simulink model "MicrogridControl"  (R2025b)
settings: Solver=VariableStepAuto  StartTime=0.0  StopTime=8  FixedStep=Ts  RelTol=1e-3
PreLoadFcn:
  | NormalOperation;
  | MicrogridControlParam;
undefined symbols (not defined in the file): base, bessModeInitial, bessSystem, bessVoltage, breakerStatus, DiscIntNeverNeededParam, ee_sli_rtmsupport, event, gcbh, generator, gflInverter, gfmInverter, Inertia, lineInductance, lineResistance, machine, plannedIsland, pmsm, powerLimit, powerQuality, PV, PVInverter, ref, resync, solar, solarInsolationChange, systemFrequency, Ts, windController, windSystem, windTurbine
libraries: nesl_utility x234, ee_lib x174, fl_lib x143, eeGeneralControl x137, simulink x78, eeTransforms x47, slpidlib x23, nesl_utility_internal x12, eePwmGenerator x9, eeSinusoidalMeasurementV2 x9, custom_lib x7, batteryecm_lib x6
(part 23 of 25)

== system MicrogridControl/BESS/BESS Integrated3/Detailed/BESS Controller/Grid Forming/Measurement/Frequency Measurement/Frequency Measurement/Postive Sequence ==
  abc : Inport
  Complex to Real-Imag : ComplexToRealImag
  Demux : Demux  Outputs=3
  Symmetrical-Components Transform : eeTransforms/Symmetrical-Components Transform  PowerInvariant=off
  Terminator : Terminator
  Terminator1 : Terminator
  Terminator2 : Terminator
  Transpose : Math  Operator=transpose
  posSeq : Outport
  wires:
  Demux/3 -> Terminator2/1
  Demux/2 -> Terminator1/1
  Complex to Real-Imag/2 -> Terminator/1
  abc/1 -> Transpose/1
  Demux/1 -> Complex to Real-Imag/1
  Complex to Real-Imag/1 -> posSeq/1
  Symmetrical-Components Transform/1 -> Demux/1
  Transpose/1 -> Symmetrical-Components Transform/1

== system MicrogridControl/BESS/BESS Integrated3/Detailed/BESS Controller/Grid Forming/Power Control/ActivePowerControl/vsmControl/Damping Frequency ==
  fref : Inport
  ConstantFreqReference : Subsystem  VariantControl=constFreq
  WithFrequencyMeasurement : Subsystem  VariantControl=freqMeas
  fmeas : Outport

== system MicrogridControl/BESS/BESS Integrated3/Detailed/BESS Controller/Grid Forming/Power Control/ActivePowerControl/vsmControl/Power Reference Selection ==
  cntrlflag : Inport
  Pref : Inport  Port=2
  fref : Inport  Port=3
  Wsm : Inport  Port=4
  If : If
  If Action Subsystem : Subsystem  TreatAsAtomicUnit=on
  If Action Subsystem1 : Subsystem  TreatAsAtomicUnit=on
  Merge : Merge
  Scope : Scope
      settings: ActiveDisplayYMinimum=-0.024489680768438882  ActiveDisplayYMaximum=0.022000264002839637
  power : Outport
  wires:
  Wsm/1 -> [Wsm]
  Merge/1 -> power/1, Scope/1
  cntrlflag/1 -> If/1
  If/2 -> If Action Subsystem1/Action
  If Action Subsystem/1(Power) -> Merge/1
  [Wsm] -> If Action Subsystem/2(Wsm)
  fref/1 -> If Action Subsystem1/1(fref)
  [Wsm] -> If Action Subsystem1/2(Wsm)
  Pref/1 -> If Action Subsystem/1(Pref)
  If/1 -> If Action Subsystem/Action
  If Action Subsystem1/1(Power) -> Merge/2

== system MicrogridControl/BESS/BESS Integrated3/Detailed/BESS Controller/Grid Forming/Power Control/ReactiveControl/Voltage  Reference Selection/If Action Subsystem ==
  note: Vs-delV
  Qref : Inport
  Qmeas : Inport  Port=2
  Action Port : ActionPort  ActionPortLabel=if(u1 > 0)
  Constant : Constant  Value=voltreference
  Gain : Gain  Gain=1%QVoltDroop
  Low-Pass Filter (Discrete or Continuous) : eeGeneralControl/Low-Pass Filter (Discrete or Continuous)  K=1  T=QVoltFilterTC  B=inf  A=-inf  init_option=Specify as parameter  x0=0  Ts=activePowerSampleTime
  Product1 : Product
  Scope : Scope
      settings: ActiveDisplayYMinimum=-0.48916032129163395  ActiveDisplayYMaximum=3.1082432095983168
  Scope1 : Scope  NumInputPorts=2
      settings: ActiveDisplayYMinimum=-1.3317089011874013  ActiveDisplayYMaximum=1.2590787667985386  DataLoggingVariableName=ScopeData5
  Sum : Sum  Inputs=|+-
  Sum1 : Sum  Inputs=|++
  Vd : Outport
  wires:
  Product1/1 -> Vd/1  "V"
  Sum1/1 -> Product1/1
  Sum/1 -> Gain/1
  Low-Pass Filter (Discrete or Continuous)/1 -> Sum/2
  Qref/1 -> Scope1/1, Sum/1
  Gain/1 -> Sum1/1, Scope/1
  Qmeas/1 -> Scope1/2, Low-Pass Filter (Discrete or Continuous)/1
  Constant/1 -> Sum1/2, Product1/2

== system MicrogridControl/BESS/BESS Integrated3/Detailed/BESS Controller/Grid Forming/Power Control/ReactiveControl/Voltage  Reference Selection/If Action Subsystem1 ==
  note: Vs-delV
  Vref : Inport
  Vmeas : Inport  Port=2
  Action Port : ActionPort  ActionPortLabel=else
  Constant : Constant  Value=voltreference+0.05
  Gain : Gain  Gain=2%2/QVoltDroop
  Low-Pass Filter (Discrete or Continuous) : eeGeneralControl/Low-Pass Filter (Discrete or Continuous)  K=1  T=QVoltFilterTC  B=inf  A=-inf  init_option=Specify as parameter  x0=0  Ts=activePowerSampleTime
  Product1 : Product
  Scope : Scope
      settings: ActiveDisplayYMinimum=0.18931616111927707  ActiveDisplayYMaximum=6.6456315376534141  DataLoggingVariableName=ScopeData11  DataLoggingSaveFormat=Array
  Scope1 : Scope
      settings: ActiveDisplayYMinimum=-0.70570607622731063  ActiveDisplayYMaximum=1.2282506152075161  DataLoggingVariableName=ScopeData12  DataLoggingSaveFormat=Array
  Scope2 : Scope  NumInputPorts=2
      settings: ActiveDisplayYMinimum=-1  ActiveDisplayYMaximum=1  DataLoggingVariableName=ScopeData13  DataLoggingSaveFormat=Array
  Sum : Sum  Inputs=|+-
  Sum1 : Sum  Inputs=|++
  Voltage : Outport
  wires:
  Sum1/1 -> Product1/2
  Product1/1 -> Scope/1, Voltage/1  "V"
  Sum/1 -> Gain/1
  Low-Pass Filter (Discrete or Continuous)/1 -> Scope1/1, Sum/2
  Constant/1 -> Sum1/2
  Vmeas/1 -> Low-Pass Filter (Discrete or Continuous)/1, Scope2/2
  Gain/1 -> Sum1/1
  Vref/1 -> Sum/1, Product1/1, Scope2/1

== system MicrogridControl/Solar/Solar Plant Integrated/Detailed/PV Plant & Controller/Controller/MPPT/Solar PV Controller/DC voltage controller & current reference/Current limits ==
  Imax : Inport
  idref : Inport  Port=2
  Sqrt1 : Sqrt
  Square3 : Math  Operator=square
  Square4 : Math  Operator=square
  Sum9 : Sum  Inputs=|+-
  iubd : Outport
  iubq : Outport  Port=2
  wires:
  idref/1 -> Square4/1
  Sqrt1/1 -> iubq/1
  Imax/1 -> Square3/1, iubd/1
  Square4/1 -> Sum9/2
  Square3/1 -> Sum9/1
  Sum9/1 -> Sqrt1/1

== system MicrogridControl/Solar/Solar Plant Integrated/Detailed/PV Plant & Controller/Controller/MPPT/Solar PV Controller/DC voltage controller & current reference/If Action Subsystem ==
  note: id_ref_generator
  note: iq_ref_generator
  Q ref : Inport
  Vmag : Inport  Port=2
  P pv : Inport  Port=3
  vdc : Inport  Port=4
  vdc ref : Inport  Port=5
  Action Port : ActionPort
  Subsystem : Subsystem
  Subsystem1 : Subsystem
  iq ref : Outport
  id ref : Outport  Port=2
  wires:
  Subsystem/1(iqref) -> iq ref/1
  Subsystem1/1(idref) -> id ref/1
  vdc ref/1 -> Subsystem1/4(vdc ref)
  Vmag/1 -> Subsystem/1(V mag), Subsystem1/1(Vmag)
  vdc/1 -> Subsystem1/3(vdc)
  Q ref/1 -> Subsystem/3(Q ref)
  P pv/1 -> Subsystem1/2(P pv)
  [ubiq] -> Subsystem/2(iq ub)
  [ubid] -> Subsystem1/5(id ub)

== system MicrogridControl/Solar/Solar Plant Integrated/Detailed/PV Plant & Controller/Controller/MPPT/Solar PV Controller/DC voltage controller & current reference/Subsystem ==
  V mag : Inport
  iq ub : Inport  Port=2
  Q ref : Inport  Port=3
  Constant : Constant  Value=1e-3
  Data Type Conversion Inherited : simulink/Signal Attributes/Data Type Conversion Inherited  ConvertRealWorld=Real World Value  DoSatur=off
  Divide2 : Product  Inputs=*/
  Gain1 : Gain  Gain=-1
  Gain3 : Gain  Gain=-1
  Saturation Dynamic2 : simulink/Discontinuities/Saturation Dynamic  OutMin=[]  OutMax=[]  OutDataTypeStr=Inherit: Same as second input  OutDataType=fixdt(1, 16)  OutScaling=2^-10  DoSatur=off
  Scope : Scope  NumInputPorts=3
      settings: ActiveDisplayYMinimum=-1  ActiveDisplayYMaximum=1  DataLoggingVariableName=ScopeData8
  Switch : Switch  Criteria=u2 ~= 0  SaturateOnIntegerOverflow=off  InputSameDT=off
  iq ub1 : InportShadow  Port=2
  iqref : Outport
  wires:
  Gain1/1 -> iqref/1
  Data Type Conversion Inherited/1 -> Switch/3
  Constant/1 -> Data Type Conversion Inherited/2
  Switch/1 -> Divide2/2
  V mag/1 -> Switch/1, Switch/2, Data Type Conversion Inherited/1
  Saturation Dynamic2/1 -> Gain1/1
  iq ub/1 -> Scope/1, Saturation Dynamic2/1
  Gain3/1 -> Scope/3, Saturation Dynamic2/3
  Q ref/1 -> Divide2/1
  Divide2/1 -> Scope/2, Saturation Dynamic2/2
  iq ub1/1 -> Gain3/1

== system MicrogridControl/Solar/Solar Plant Integrated/Detailed/PV Plant & Controller/Controller/MPPT/Solar PV Controller/DC voltage controller & current reference/Subsystem1 ==
  Vmag : Inport
  P pv : Inport  Port=2
  vdc : Inport  Port=3
  vdc ref : Inport  Port=4
  id ub : Inport  Port=5
  Constant : Constant  Value=1e-3
  Constant4 : Constant  Value=0
  Data Type Conversion Inherited : simulink/Signal Attributes/Data Type Conversion Inherited  ConvertRealWorld=Real World Value  DoSatur=off
  Divide : Product  Inputs=/*
  Gain4 : Gain  Gain=1/(mVAbase)
  Saturation Dynamic1 : simulink/Discontinuities/Saturation Dynamic  OutMin=[]  OutMax=[]  OutDataTypeStr=Inherit: Same as second input  OutDataType=fixdt(1, 16)  OutScaling=2^-10  DoSatur=off
  Scope : Scope  NumInputPorts=2
      settings: ActiveDisplayYMinimum=961.255553355759  ActiveDisplayYMaximum=1181.2786383151777
  Scope1 : Scope  NumInputPorts=3
      settings: ActiveDisplayYMinimum=-1  ActiveDisplayYMaximum=1  DataLoggingVariableName=ScopeData7
  Sum : Sum  Inputs=|++
  Switch : Switch  Criteria=u2 ~= 0  SaturateOnIntegerOverflow=off  InputSameDT=off
  V_dc_Controller1 : Subsystem
  idref : Outport
  wires:
  Data Type Conversion Inherited/1 -> Switch/3
  Constant/1 -> Data Type Conversion Inherited/2
  Switch/1 -> Divide/1
  Vmag/1 -> Switch/1, Switch/2, Data Type Conversion Inherited/1
  vdc/1 -> Scope/1, V_dc_Controller1/1(vdc)
  Saturation Dynamic1/1 -> Scope1/3, idref/1
  Divide/1 -> Sum/1
  Gain4/1 -> Divide/2
  id ub/1 -> Saturation Dynamic1/1, Scope1/1
  vdc ref/1 -> Scope/2, V_dc_Controller1/2(vdc ref)
  Sum/1 -> Scope1/2, Saturation Dynamic1/2
  V_dc_Controller1/1(Out1) -> Sum/2
  P pv/1 -> Gain4/1
  Constant4/1 -> Saturation Dynamic1/3

== system MicrogridControl/Solar/Solar Plant Integrated/Detailed/PV Plant & Controller/Controller/MPPT/Solar PV Controller/PLL & Measurements/Subsystem ==
  abc : Inport
  Demux : Demux  Outputs=3
  Park Transform : eeTransforms/Park Transform  AxisAlignment=Q-axis  PowerInvariant=off
  "Sinusoidal Measurement (PLL, Three-Phase)" : eeSinusoidalMeasurementV2/Sinusoidal Measurement (PLL, Three-Phase)  InputFilter=on  InputNormalization=off  Kp_LF=Kppll  Ki_LF=Kipll  F0=frequency  Theta0=initialPhase  Ts=sampleTime
  Terminator : Terminator
  mag : Outport
  freq : Outport  Port=2
  angle : Outport  Port=3
  Vd : Outport  Port=4
  Vq : Outport  Port=5
  wires:
  "Sinusoidal Measurement (PLL, Three-Phase)"/3 -> mag/1
  "Sinusoidal Measurement (PLL, Three-Phase)"/1 -> freq/1
  Demux/2 -> Vq/1
  Demux/1 -> Vd/1
  Park Transform/1 -> Demux/1
  abc/1 -> "Sinusoidal Measurement (PLL, Three-Phase)"/1, Park Transform/1
  Demux/3 -> Terminator/1
  "Sinusoidal Measurement (PLL, Three-Phase)"/2 -> Park Transform/2, angle/1

== system MicrogridControl/Solar/Solar Plant Integrated/Detailed/PV Plant & Controller/Controller/MPPT/Solar PV Controller/Variant Subsystem/INC MPP ==
  Ipv : Inport
  Vpv : Inport  Port=2
  Abs : Abs  SaturateOnIntegerOverflow=off
  Add : Sum
  Constant : Constant  Value=0  SampleTime=sampleTime
  Constant1 : Constant  Value=delV  SampleTime=sampleTime
  Data Type Conversion Inherited : simulink/Signal Attributes/Data Type Conversion Inherited  ConvertRealWorld=Real World Value  DoSatur=off
  Data Type Conversion Inherited1 : simulink/Signal Attributes/Data Type Conversion Inherited  ConvertRealWorld=Real World Value  DoSatur=off
  Divide : Product  Inputs=*/
  Divide1 : Product  Inputs=*/
  Filtered Derivative (Discrete or Continuous) : eeGeneralControl/Filtered Derivative (Discrete or Continuous)  K=1  T=tSettling*2  B=inf  A=-inf  minRatio=1  init_option=Inherited from block input  x0=0  Ts=sampleTime
  Filtered Derivative (Discrete or Continuous)1 : eeGeneralControl/Filtered Derivative (Discrete or Continuous)  K=1  T=tSettling*2  B=inf  A=-inf  minRatio=1  init_option=Inherited from block input  x0=0  Ts=sampleTime
  Subtract5 : Sum  Inputs=-+
  Sum2 : Sum  Inputs=|++
  Switch : Switch  Criteria=u2 ~= 0  SaturateOnIntegerOverflow=off  InputSameDT=off
  Switch1 : Switch  Criteria=u2 > Threshold  SaturateOnIntegerOverflow=off  InputSameDT=off
  Switch4 : Switch  Criteria=u2 > Threshold  Threshold=1e-2  SaturateOnIntegerOverflow=off  InputSameDT=off
  Switch5 : Switch  Criteria=u2 > Threshold  SaturateOnIntegerOverflow=off  InputSameDT=off
  start MPPT Voltage : Constant  Value=Vdc  SampleTime=sampleTime
  Vmpp : Outport  VectorParamsAs1DForOutWhenUnconnected=off
  wires:
  Data Type Conversion Inherited1/1 -> Subtract5/1, Add/2
  Switch4/1 -> Data Type Conversion Inherited1/2
  start MPPT Voltage/1 -> Data Type Conversion Inherited/2
  Data Type Conversion Inherited/1 -> Switch5/3
  Switch1/1 -> Vmpp/1
  Constant1/1 -> Switch4/1
  Constant/1 -> Switch4/3
  Abs/1 -> Switch4/2
  Filtered Derivative (Discrete or Continuous)1/1 -> Divide/2, Switch/2
  [Vdec] -> Switch1/3
  [Vinc] -> Switch1/1
  Switch/1 -> Abs/1, Switch1/2
  Sum2/1 -> Switch/1
  Divide1/1 -> Sum2/2
  Divide/1 -> Sum2/1
  Filtered Derivative (Discrete or Continuous)/1 -> Divide/1, Switch/3
  Subtract5/1 -> [Vdec]  "DEC"
  Add/1 -> [Vinc]  "INC"
  Vpv/1 -> Switch5/1, Switch5/2, Data Type Conversion Inherited/1, Divide1/2, Filtered Derivative (Discrete or Continuous)1/1
  Switch5/1 -> Subtract5/2, Add/1, Data Type Conversion Inherited1/1
  Ipv/1 -> Divide1/1, Filtered Derivative (Discrete or Continuous)/1

== system MicrogridControl/Solar/Solar Plant Integrated/Detailed/PV Plant & Controller/Controller/MPPT/Solar PV Controller/Variant Subsystem/P&O MPP ==
  Ipv : Inport
  Vpv : Inport  Port=2
  AND1 : Logic  IconShape=distinctive  AllPortsSameDT=off  OutDataTypeStr=boolean
  Add : Sum
  Compare To Zero1 : simulink/Logic and Bit Operations/Compare To Zero  relop=>=  OutDataTypeStr=boolean
  Compare To Zero2 : simulink/Logic and Bit Operations/Compare To Zero  relop=>=  OutDataTypeStr=boolean
  Constant1 : Constant  Value=delV  SampleTime=sampleTime
  Data Type Conversion Inherited : simulink/Signal Attributes/Data Type Conversion Inherited  ConvertRealWorld=Real World Value  DoSatur=off
  Data Type Conversion Inherited1 : simulink/Signal Attributes/Data Type Conversion Inherited  ConvertRealWorld=Real World Value  DoSatur=off
  Filtered Derivative (Discrete or Continuous) : eeGeneralControl/Filtered Derivative (Discrete or Continuous)  K=1  T=tSettling*2  B=inf  A=-inf  minRatio=1  init_option=Inherited from block input  x0=0  Ts=sampleTime
  Filtered Derivative (Discrete or Continuous)1 : eeGeneralControl/Filtered Derivative (Discrete or Continuous)  K=1  T=tSettling*2  B=inf  A=-inf  minRatio=1  init_option=Inherited from block input  x0=0  Ts=sampleTime
  NOR : Logic  Operator=NOR  IconShape=distinctive  AllPortsSameDT=off  OutDataTypeStr=boolean
  OR : Logic  Operator=OR  IconShape=distinctive  AllPortsSameDT=off  OutDataTypeStr=boolean
  Product : Product
  Subtract5 : Sum  Inputs=-+
  Switch4 : Switch  Criteria=u2 ~= 0  SaturateOnIntegerOverflow=off  InputSameDT=off
  Switch5 : Switch  Criteria=u2 > Threshold  SaturateOnIntegerOverflow=off  InputSameDT=off
  start MPPT Voltage : Constant  Value=Vdc  SampleTime=sampleTime
  Vmpp : Outport  VectorParamsAs1DForOutWhenUnconnected=off
  wires:
  Data Type Conversion Inherited1/1 -> Subtract5/1, Add/2
  start MPPT Voltage/1 -> Data Type Conversion Inherited/2
  Data Type Conversion Inherited/1 -> Switch5/3
  Switch4/1 -> Vmpp/1
  Product/1 -> Filtered Derivative (Discrete or Continuous)/1
  Ipv/1 -> Product/1
  [Vinc] -> Switch4/1
  AND1/1 -> OR/1
  Filtered Derivative (Discrete or Continuous)/1 -> Compare To Zero2/1
  Filtered Derivative (Discrete or Continuous)1/1 -> Compare To Zero1/1
  [Vdec] -> Switch4/3
  Subtract5/1 -> [Vdec]  "DEC"
  NOR/1 -> OR/2
  Add/1 -> [Vinc]  "INC"
  Vpv/1 -> Switch5/1, Switch5/2, Data Type Conversion Inherited/1, Filtered Derivative (Discrete or Continuous)1/1, Product/2
  Constant1/1 -> Data Type Conversion Inherited1/2
  Switch5/1 -> Subtract5/2, Add/1, Data Type Conversion Inherited1/1
  Compare To Zero2/1 -> AND1/1, NOR/2
  Compare To Zero1/1 -> AND1/2, NOR/1
  OR/1 -> Switch4/2

== system MicrogridControl/Solar/Solar Plant Integrated/Detailed/PV Plant & Controller/Controller/Power Reference/Power Reference Controller/PLL & Measurements/Measurement1 ==
  u : Inport
  Lead-Lag (Discrete or Continuous) : eeGeneralControl/Lead-Lag (Discrete or Continuous)  T1=0  T2=1e-3  B=inf  A=-inf  init_option=Inherited from block input  x0=0  Ts=Ts
  Vg : Outport
  wires:
  u/1 -> Lead-Lag (Discrete or Continuous)/1
  Lead-Lag (Discrete or Continuous)/1 -> Vg/1

== system MicrogridControl/Solar/Solar Plant Integrated/Detailed/PV Plant & Controller/Controller/Power Reference/Power Reference Controller/PLL & Measurements/Measurement2 ==
  u : Inport
  Lead-Lag (Discrete or Continuous) : eeGeneralControl/Lead-Lag (Discrete or Continuous)  T1=0  T2=1e-3  B=inf  A=-inf  init_option=Inherited from block input  x0=0  Ts=Ts
  Vg : Outport
  wires:
  u/1 -> Lead-Lag (Discrete or Continuous)/1
  Lead-Lag (Discrete or Continuous)/1 -> Vg/1

== system MicrogridControl/Solar/Solar Plant Integrated/Detailed/PV Plant & Controller/Controller/Power Reference/Power Reference Controller/PLL & Measurements/Subsystem ==
  Vabc : Inport
  Iabc : Inport  Port=2
  Demux : Demux  Outputs=3
  Demux1 : Demux  Outputs=3
  Park Transform : eeTransforms/Park Transform  AxisAlignment=Q-axis  PowerInvariant=off
  Park Transform1 : eeTransforms/Park Transform  AxisAlignment=Q-axis  PowerInvariant=off
  Scope : Scope  NumInputPorts=2
      settings: ActiveDisplayYMinimum=0.97158  ActiveDisplayYMaximum=1.00612  DataLoggingVariableName=ScopeData5
  "Sinusoidal Measurement (PLL, Three-Phase)" : eeSinusoidalMeasurementV2/Sinusoidal Measurement (PLL, Three-Phase)  InputFilter=on  InputNormalization=off  Kp_LF=kpPLL  Ki_LF=kiPLL  F0=frequency  Theta0=0  Ts=-1
  Terminator : Terminator
  Terminator1 : Terminator
  mag : Outport
  freq : Outport  Port=2
  angle : Outport  Port=3
  Vd : Outport  Port=4
  Vq : Outport  Port=5
  Id1 : Outport  Port=6
  Iq1 : Outport  Port=7
  wires:
  Iabc/1 -> Park Transform1/1
  Demux1/3 -> Terminator1/1
  Demux1/2 -> Iq1/1
  Demux1/1 -> Id1/1
  Park Transform1/1 -> Demux1/1
  "Sinusoidal Measurement (PLL, Three-Phase)"/3 -> mag/1
  "Sinusoidal Measurement (PLL, Three-Phase)"/1 -> freq/1
  "Sinusoidal Measurement (PLL, Three-Phase)"/2 -> Park Transform/2, Park Transform1/2, angle/1
  Demux/2 -> Vq/1, Scope/2
  Demux/1 -> Vd/1, Scope/1
  Park Transform/1 -> Demux/1
  Vabc/1 -> "Sinusoidal Measurement (PLL, Three-Phase)"/1, Park Transform/1
  Demux/3 -> Terminator/1

== system MicrogridControl/Solar/Solar Plant Integrated/Detailed/PV Plant & Controller/Controller/Power Reference/Power Reference Controller/Power Reference Controller/Current_controller ==
  id-ref : Inport
  ipvd : Inport  Port=2
  iqref : Inport  Port=3
  iq : Inport  Port=4
  Vd : Inport  Port=5
  Vq : Inport  Port=6
  Constant4 : Constant  Value=0
  Gain1 : Gain  Gain=2*1*pi*60*L/zbase
  Gain2 : Gain  Gain=2*1*pi*60*L/zbase
  Mux1 : Mux  Inputs=3
  PID Controller : slpidlib/PID Controller  Controller=PID  Form=Parallel  TimeDomain=Discrete-time  UseExternalTs=off  SampleTime=-1  IntegratorMethod=Forward Euler  FilterMethod=Forward Euler  ControllerParametersSource=internal  P=Kpic  I=Kiic  UseKiTs=off  D=Kd  UseExternalDerivativeSource=off  N=100  UseFilter=on  TunerSelectOption=Transfer Function Based (PID Tuner App)  InitialConditionSource=internal  InitialConditionForIntegrator=0  InitialConditionForFilter=0  DifferentiatorICPrevScaledInput=0  ExternalReset=none  TrackingMode=off  Kt=1  LimitOutput=on  SatLimitsSource=internal  UpperSaturationLimit=3  LowerSaturationLimit=-3  LinearizeAsGain=on  AntiWindupMode=clamping  Kb=1  LimitIntegrator=on  UpperIntegratorSaturationLimit=3  LowerIntegratorSaturationLimit=-3  POutMin=[]  POutMax=[]  IOutMin=[]  IOutMax=[]  DOutMin=[]  DOutMax=[]  NOutMin=[]  NOutMax=[]  SumOutMin=[]  SumOutMax=[]  SaturationOutMin=[]  SaturationOutMax=[]  PParamMin=[]  PParamMax=[]  IParamMin=[]  IParamMax=[]  DParamMin=[]  DParamMax=[]  NParamMin=[]  NParamMax=[]  KbParamMin=[]  KbParamMax=[]  KtParamMin=[]  KtParamMax=[]  KbOutMin=[]  KbOutMax=[]  KtOutMin=[]  KtOutMax=[]  IntegratorOutMin=[]  IntegratorOutMax=[]  FilterOutMin=[]  FilterOutMax=[]  SumI1OutMin=[]  SumI1OutMax=[]  SumI2OutMin=[]  SumI2OutMax=[]  SumI3OutMin=[]  SumI3OutMax=[]  SumI4OutMin=[]  SumI4OutMax=[]  SumDOutMin=[]  SumDOutMax=[]  DifferentiatorOutMin=[]  DifferentiatorOutMax=[]  FilterDiffOutCoefMin=[]  FilterDiffOutCoefMax=[]  ReciprocalOutMin=[]  ReciprocalOutMax=[]  SumDenOutMin=[]  SumDenOutMax=[]  SumNumOutMin=[]  SumNumOutMax=[]  DivideOutMin=[]  DivideOutMax=[]  UdiffTsProdOutMin=[]  UdiffTsProdOutMax=[]  NTsProdOutMin=[]  NTsProdOutMax=[]  UintegralTsProdOutMin=[]  UintegralTsProdOutMax=[]  UngainTsProdOutMin=[]  UngainTsProdOutMax=[]  ClampingZeroOutDataTypeStr=Inherit: Inherit via back propagation  ClampingZeroOutMin=[]  ClampingZeroOutMax=[]  FilterDenConstantOutDataTypeStr=Inherit: Inherit via back propagation  FilterDenConstantOutMin=[]  FilterDenConstantOutMax=[]  PCopyOutDataTypeStr=Inherit: Inherit via back propagation  PCopyOutMin=[]  PCopyOutMax=[]  NCopyOutDataTypeStr=Inherit: Inherit via back propagation  NCopyOutMin=[]  NCopyOutMax=[]  IntegratorContinuousStateAttributes=''  IntegratorStateMustResolveToSignalObject=off  IntegratorRTWStateStorageClass=Auto  FilterContinuousStateAttributes=''  FilterStateMustResolveToSignalObject=off  FilterRTWStateStorageClass=Auto  ParallelPVariant=InternalParameters  IdealPVariant=Disabled  IVariant=InternalParameters  DVariant=InternalParameters  IntegratorVariant=Discrete  SatVariant=Enabled  AWVariant=DiscClampingParallel  PCopyVariant=Disabled  TRVariant=Disabled  FdbkBlocksVariant=Forward  IdealPFdbkVariant=Disabled  SatFdbkVariant=Disabled  DerivativeFilterVariant=ForwardEulerFilter  NVariant=InternalParameters  NCopyVariant=Disabled  FilterICVariant=InternalICsFilter  IntegratorICVariant=InternalICs  ExternalResetVariant=Disabled  TRSumVariant=Passthrough  SumFdbkVariant=Disabled  SumVariant=Sum_PID  TsampFilterVariant=InternalTs  TsampNgainVariant=Passthrough  TsampIntegralVariant=Disabled_SignalSpec  ExternalSaturationOutDataTypeStr=Inherit: Same as second input  DerivativeSourceVariant=ErrorSignal  PreIntVariant=InternalPreInt
  PID Controller1 : slpidlib/PID Controller  Controller=PID  Form=Parallel  TimeDomain=Discrete-time  UseExternalTs=off  SampleTime=-1  IntegratorMethod=Forward Euler  FilterMethod=Forward Euler  ControllerParametersSource=internal  P=Kpic  I=Kiic  UseKiTs=off  D=Kd  UseExternalDerivativeSource=off  N=100  UseFilter=on  TunerSelectOption=Transfer Function Based (PID Tuner App)  InitialConditionSource=internal  InitialConditionForIntegrator=0  InitialConditionForFilter=0  DifferentiatorICPrevScaledInput=0  ExternalReset=none  TrackingMode=off  Kt=1  LimitOutput=on  SatLimitsSource=internal  UpperSaturationLimit=3  LowerSaturationLimit=-3  LinearizeAsGain=on  AntiWindupMode=clamping  Kb=1  LimitIntegrator=on  UpperIntegratorSaturationLimit=3  LowerIntegratorSaturationLimit=-3  POutMin=[]  POutMax=[]  IOutMin=[]  IOutMax=[]  DOutMin=[]  DOutMax=[]  NOutMin=[]  NOutMax=[]  SumOutMin=[]  SumOutMax=[]  SaturationOutMin=[]  SaturationOutMax=[]  PParamMin=[]  PParamMax=[]  IParamMin=[]  IParamMax=[]  DParamMin=[]  DParamMax=[]  NParamMin=[]  NParamMax=[]  KbParamMin=[]  KbParamMax=[]  KtParamMin=[]  KtParamMax=[]  KbOutMin=[]  KbOutMax=[]  KtOutMin=[]  KtOutMax=[]  IntegratorOutMin=[]  IntegratorOutMax=[]  FilterOutMin=[]  FilterOutMax=[]  SumI1OutMin=[]  SumI1OutMax=[]  SumI2OutMin=[]  SumI2OutMax=[]  SumI3OutMin=[]  SumI3OutMax=[]  SumI4OutMin=[]  SumI4OutMax=[]  SumDOutMin=[]  SumDOutMax=[]  DifferentiatorOutMin=[]  DifferentiatorOutMax=[]  FilterDiffOutCoefMin=[]  FilterDiffOutCoefMax=[]  ReciprocalOutMin=[]  ReciprocalOutMax=[]  SumDenOutMin=[]  SumDenOutMax=[]  SumNumOutMin=[]  SumNumOutMax=[]  DivideOutMin=[]  DivideOutMax=[]  UdiffTsProdOutMin=[]  UdiffTsProdOutMax=[]  NTsProdOutMin=[]  NTsProdOutMax=[]  UintegralTsProdOutMin=[]  UintegralTsProdOutMax=[]  UngainTsProdOutMin=[]  UngainTsProdOutMax=[]  ClampingZeroOutDataTypeStr=Inherit: Inherit via back propagation  ClampingZeroOutMin=[]  ClampingZeroOutMax=[]  FilterDenConstantOutDataTypeStr=Inherit: Inherit via back propagation  FilterDenConstantOutMin=[]  FilterDenConstantOutMax=[]  PCopyOutDataTypeStr=Inherit: Inherit via back propagation  PCopyOutMin=[]  PCopyOutMax=[]  NCopyOutDataTypeStr=Inherit: Inherit via back propagation  NCopyOutMin=[]  NCopyOutMax=[]  IntegratorContinuousStateAttributes=''  IntegratorStateMustResolveToSignalObject=off  IntegratorRTWStateStorageClass=Auto  FilterContinuousStateAttributes=''  FilterStateMustResolveToSignalObject=off  FilterRTWStateStorageClass=Auto  ParallelPVariant=InternalParameters  IdealPVariant=Disabled  IVariant=InternalParameters  DVariant=InternalParameters  IntegratorVariant=Discrete  SatVariant=Enabled  AWVariant=DiscClampingParallel  PCopyVariant=Disabled  TRVariant=Disabled  FdbkBlocksVariant=Forward  IdealPFdbkVariant=Disabled  SatFdbkVariant=Disabled  DerivativeFilterVariant=ForwardEulerFilter  NVariant=InternalParameters  NCopyVariant=Disabled  FilterICVariant=InternalICsFilter  IntegratorICVariant=InternalICs  ExternalResetVariant=Disabled  TRSumVariant=Passthrough  SumFdbkVariant=Disabled  SumVariant=Sum_PID  TsampFilterVariant=InternalTs  TsampNgainVariant=Passthrough  TsampIntegralVariant=Disabled_SignalSpec  ExternalSaturationOutDataTypeStr=Inherit: Same as second input  DerivativeSourceVariant=ErrorSignal  PreIntVariant=InternalPreInt
  Saturation : Saturate  UpperLimit=1.2  LowerLimit=-1.2
  Saturation1 : Saturate  UpperLimit=1.2  LowerLimit=-1.2
  Scope : Scope  NumInputPorts=2
      settings: ActiveDisplayYMinimum=0.49995  ActiveDisplayYMaximum=0.50039
  Scope1 : Scope  NumInputPorts=2
      settings: ActiveDisplayYMinimum=-1  ActiveDisplayYMaximum=1  DataLoggingVariableName=ScopeData2
  Scope2 : Scope  NumInputPorts=3
      settings: ActiveDisplayYMinimum=0.92426  ActiveDisplayYMaximum=1.0261  DataLoggingVariableName=ScopeData2
  Sum1 : Sum  Inputs=|+-
  Sum3 : Sum  Inputs=|++-
  Sum4 : Sum  Inputs=|+++
  Sum5 : Sum  Inputs=|+-
  mdq0 : Outport
  wires:
  Vd/1 -> Sum3/1, Scope2/1
  Saturation1/1 -> Mux1/2
  Saturation/1 -> Mux1/1
  iqref/1 -> Sum5/1, Scope1/1
  Mux1/1 -> mdq0/1
  Sum4/1 -> [Eq], Saturation1/1
  PID Controller1/1 -> Sum4/1
  Sum5/1 -> PID Controller1/1
  Constant4/1 -> Mux1/3
  Sum1/1 -> PID Controller/1
  iq/1 -> Sum5/2, Gain2/1, Scope1/2
  Vq/1 -> Sum4/2
  Gain1/1 -> Sum4/3
  id-ref/1 -> Sum1/1, Scope/1
  ipvd/1 -> Sum1/2, Gain1/1, Scope/2
  Gain2/1 -> Sum3/3, Scope2/3
  Sum3/1 -> [Ed], Saturation/1
  PID Controller/1 -> Sum3/2, Scope2/2

== system MicrogridControl/Solar/Solar Plant Integrated/Detailed/PV Plant & Controller/Controller/Power Reference/Power Reference Controller/Power Reference Controller/Reference Current ==
  note: Avoid division by zero during start
  note: Current Limiters
  V-mag : Inport
  LVRT_iq : Inport  Port=2
  PRef : Inport  Port=3
  QRef : Inport  Port=4
  Constant1 : Constant
  Constant3 : Constant  Value=Imax
  Current limits : Subsystem
  Refernce id generation : Subsystem
  Refernce iq generation : Subsystem
  Switch : Switch  Criteria=u2 ~= 0  SaturateOnIntegerOverflow=off  InputSameDT=off
  Unit Delay1 : UnitDelay  SampleTime=Ts  HasFrameUpgradeWarning=on
  Unit Delay3 : UnitDelay  SampleTime=Ts  HasFrameUpgradeWarning=on
  id_ref : Outport
  iq_ref : Outport  Port=2
  wires:
  Current limits/2(iubd) -> Refernce id generation/2(ubid)
  PRef/1 -> Refernce id generation/3(PRef)
  QRef/1 -> Refernce iq generation/4(Q_ref)
  Constant1/1 -> Switch/3
  Switch/1 -> Refernce iq generation/2(V_mag), Refernce id generation/1(V_mag)
  V-mag/1 -> Switch/2, Switch/1
  LVRT_iq/1 -> Refernce iq generation/3(LVRT_iq)
  Refernce iq generation/1(iq_ref) -> iq_ref/1, Unit Delay1/1
  Refernce id generation/1(id_ref) -> Unit Delay3/1, id_ref/1
  Constant3/1 -> Current limits/1(Imax)
  Unit Delay3/1 -> Current limits/3(idref)
  Current limits/1(iubq) -> Refernce iq generation/1(ubiq)
  Unit Delay1/1 -> Current limits/2(iqref)

== system MicrogridControl/Solar/Solar Plant Integrated1/Detailed/PV Plant & Controller/Controller/MPPT/Solar PV Controller/DC voltage controller & current reference/Current limits ==
  Imax : Inport
  idref : Inport  Port=2
  Sqrt1 : Sqrt
  Square3 : Math  Operator=square
  Square4 : Math  Operator=square
  Sum9 : Sum  Inputs=|+-
  iubd : Outport
  iubq : Outport  Port=2
  wires:
  idref/1 -> Square4/1
  Sqrt1/1 -> iubq/1
  Imax/1 -> Square3/1, iubd/1
  Square4/1 -> Sum9/2
  Square3/1 -> Sum9/1
  Sum9/1 -> Sqrt1/1

== system MicrogridControl/Solar/Solar Plant Integrated1/Detailed/PV Plant & Controller/Controller/MPPT/Solar PV Controller/DC voltage controller & current reference/If Action Subsystem ==
  note: id_ref_generator
  note: iq_ref_generator
  Q ref : Inport
  Vmag : Inport  Port=2
  P pv : Inport  Port=3
  vdc : Inport  Port=4
  vdc ref : Inport  Port=5
  Action Port : ActionPort
  Subsystem : Subsystem
  Subsystem1 : Subsystem
  iq ref : Outport
  id ref : Outport  Port=2
  wires:
  Subsystem/1(iqref) -> iq ref/1
  Subsystem1/1(idref) -> id ref/1
  vdc ref/1 -> Subsystem1/4(vdc ref)
  Vmag/1 -> Subsystem/1(V mag), Subsystem1/1(Vmag)
  vdc/1 -> Subsystem1/3(vdc)
  Q ref/1 -> Subsystem/3(Q ref)
  P pv/1 -> Subsystem1/2(P pv)
  [ubiq] -> Subsystem/2(iq ub)
  [ubid] -> Subsystem1/5(id ub)

== system MicrogridControl/Solar/Solar Plant Integrated1/Detailed/PV Plant & Controller/Controller/MPPT/Solar PV Controller/DC voltage controller & current reference/Subsystem ==
  V mag : Inport
  iq ub : Inport  Port=2
  Q ref : Inport  Port=3
  Constant : Constant  Value=1e-3
  Data Type Conversion Inherited : simulink/Signal Attributes/Data Type Conversion Inherited  ConvertRealWorld=Real World Value  DoSatur=off
  Divide2 : Product  Inputs=*/
  Gain1 : Gain  Gain=-1
  Gain3 : Gain  Gain=-1
  Saturation Dynamic2 : simulink/Discontinuities/Saturation Dynamic  OutMin=[]  OutMax=[]  OutDataTypeStr=Inherit: Same as second input  OutDataType=fixdt(1, 16)  OutScaling=2^-10  DoSatur=off
  Scope : Scope  NumInputPorts=3
      settings: ActiveDisplayYMinimum=-1  ActiveDisplayYMaximum=1  DataLoggingVariableName=ScopeData8
  Switch : Switch  Criteria=u2 ~= 0  SaturateOnIntegerOverflow=off  InputSameDT=off
  iq ub1 : InportShadow  Port=2
  iqref : Outport
  wires:
  Gain1/1 -> iqref/1
  Data Type Conversion Inherited/1 -> Switch/3
  Constant/1 -> Data Type Conversion Inherited/2
  Switch/1 -> Divide2/2
  V mag/1 -> Switch/1, Switch/2, Data Type Conversion Inherited/1
  Saturation Dynamic2/1 -> Gain1/1
  iq ub/1 -> Scope/1, Saturation Dynamic2/1
  Gain3/1 -> Scope/3, Saturation Dynamic2/3
  Q ref/1 -> Divide2/1
  Divide2/1 -> Scope/2, Saturation Dynamic2/2
  iq ub1/1 -> Gain3/1

== system MicrogridControl/Solar/Solar Plant Integrated1/Detailed/PV Plant & Controller/Controller/MPPT/Solar PV Controller/DC voltage controller & current reference/Subsystem1 ==
  Vmag : Inport
  P pv : Inport  Port=2
  vdc : Inport  Port=3
  vdc ref : Inport  Port=4
  id ub : Inport  Port=5
  Constant : Constant  Value=1e-3
  Constant4 : Constant  Value=0
  Data Type Conversion Inherited : simulink/Signal Attributes/Data Type Conversion Inherited  ConvertRealWorld=Real World Value  DoSatur=off
  Divide : Product  Inputs=/*
  Gain4 : Gain  Gain=1/(mVAbase)
  Saturation Dynamic1 : simulink/Discontinuities/Saturation Dynamic  OutMin=[]  OutMax=[]  OutDataTypeStr=Inherit: Same as second input  OutDataType=fixdt(1, 16)  OutScaling=2^-10  DoSatur=off
  Scope : Scope  NumInputPorts=2
      settings: ActiveDisplayYMinimum=961.255553355759  ActiveDisplayYMaximum=1181.2786383151777
  Scope1 : Scope  NumInputPorts=3
      settings: ActiveDisplayYMinimum=-1  ActiveDisplayYMaximum=1  DataLoggingVariableName=ScopeData7
  Sum : Sum  Inputs=|++
  Switch : Switch  Criteria=u2 ~= 0  SaturateOnIntegerOverflow=off  InputSameDT=off
  V_dc_Controller1 : Subsystem
  idref : Outport
  wires:
  Data Type Conversion Inherited/1 -> Switch/3
  Constant/1 -> Data Type Conversion Inherited/2
  Switch/1 -> Divide/1
  Vmag/1 -> Switch/1, Switch/2, Data Type Conversion Inherited/1
  vdc/1 -> Scope/1, V_dc_Controller1/1(vdc)
  Saturation Dynamic1/1 -> Scope1/3, idref/1
  Divide/1 -> Sum/1
  Gain4/1 -> Divide/2
  id ub/1 -> Saturation Dynamic1/1, Scope1/1
  vdc ref/1 -> Scope/2, V_dc_Controller1/2(vdc ref)
  Sum/1 -> Scope1/2, Saturation Dynamic1/2
  V_dc_Controller1/1(Out1) -> Sum/2
  P pv/1 -> Gain4/1
  Constant4/1 -> Saturation Dynamic1/3

== system MicrogridControl/Solar/Solar Plant Integrated1/Detailed/PV Plant & Controller/Controller/MPPT/Solar PV Controller/PLL & Measurements/Subsystem ==
  abc : Inport
  Demux : Demux  Outputs=3
  Park Transform : eeTransforms/Park Transform  AxisAlignment=Q-axis  PowerInvariant=off
  "Sinusoidal Measurement (PLL, Three-Phase)" : eeSinusoidalMeasurementV2/Sinusoidal Measurement (PLL, Three-Phase)  InputFilter=on  InputNormalization=off  Kp_LF=Kppll  Ki_LF=Kipll  F0=frequency  Theta0=initialPhase  Ts=sampleTime
  Terminator : Terminator
  mag : Outport
  freq : Outport  Port=2
  angle : Outport  Port=3
  Vd : Outport  Port=4
  Vq : Outport  Port=5
  wires:
  "Sinusoidal Measurement (PLL, Three-Phase)"/3 -> mag/1
  "Sinusoidal Measurement (PLL, Three-Phase)"/1 -> freq/1
  Demux/2 -> Vq/1
  Demux/1 -> Vd/1
  Park Transform/1 -> Demux/1
  abc/1 -> "Sinusoidal Measurement (PLL, Three-Phase)"/1, Park Transform/1
  Demux/3 -> Terminator/1
  "Sinusoidal Measurement (PLL, Three-Phase)"/2 -> Park Transform/2, angle/1

== system MicrogridControl/Solar/Solar Plant Integrated1/Detailed/PV Plant & Controller/Controller/MPPT/Solar PV Controller/Variant Subsystem/INC MPP ==
  Ipv : Inport
  Vpv : Inport  Port=2
  Abs : Abs  SaturateOnIntegerOverflow=off
  Add : Sum
  Constant : Constant  Value=0  SampleTime=sampleTime
  Constant1 : Constant  Value=delV  SampleTime=sampleTime
  Data Type Conversion Inherited : simulink/Signal Attributes/Data Type Conversion Inherited  ConvertRealWorld=Real World Value  DoSatur=off
  Data Type Conversion Inherited1 : simulink/Signal Attributes/Data Type Conversion Inherited  ConvertRealWorld=Real World Value  DoSatur=off
  Divide : Product  Inputs=*/
  Divide1 : Product  Inputs=*/
  Filtered Derivative (Discrete or Continuous) : eeGeneralControl/Filtered Derivative (Discrete or Continuous)  K=1  T=tSettling*2  B=inf  A=-inf  minRatio=1  init_option=Inherited from block input  x0=0  Ts=sampleTime
  Filtered Derivative (Discrete or Continuous)1 : eeGeneralControl/Filtered Derivative (Discrete or Continuous)  K=1  T=tSettling*2  B=inf  A=-inf  minRatio=1  init_option=Inherited from block input  x0=0  Ts=sampleTime
  Subtract5 : Sum  Inputs=-+
  Sum2 : Sum  Inputs=|++
  Switch : Switch  Criteria=u2 ~= 0  SaturateOnIntegerOverflow=off  InputSameDT=off
  Switch1 : Switch  Criteria=u2 > Threshold  SaturateOnIntegerOverflow=off  InputSameDT=off
  Switch4 : Switch  Criteria=u2 > Threshold  Threshold=1e-2  SaturateOnIntegerOverflow=off  InputSameDT=off
  Switch5 : Switch  Criteria=u2 > Threshold  SaturateOnIntegerOverflow=off  InputSameDT=off
  start MPPT Voltage : Constant  Value=Vdc  SampleTime=sampleTime
  Vmpp : Outport  VectorParamsAs1DForOutWhenUnconnected=off
  wires:
  Data Type Conversion Inherited1/1 -> Subtract5/1, Add/2
  Switch4/1 -> Data Type Conversion Inherited1/2
  start MPPT Voltage/1 -> Data Type Conversion Inherited/2
  Data Type Conversion Inherited/1 -> Switch5/3
  Switch1/1 -> Vmpp/1
  Constant1/1 -> Switch4/1
  Constant/1 -> Switch4/3
  Abs/1 -> Switch4/2
  Filtered Derivative (Discrete or Continuous)1/1 -> Divide/2, Switch/2
  [Vdec] -> Switch1/3
  [Vinc] -> Switch1/1
  Switch/1 -> Abs/1, Switch1/2
  Sum2/1 -> Switch/1
  Divide1/1 -> Sum2/2
  Divide/1 -> Sum2/1
  Filtered Derivative (Discrete or Continuous)/1 -> Divide/1, Switch/3
  Subtract5/1 -> [Vdec]  "DEC"
  Add/1 -> [Vinc]  "INC"
  Vpv/1 -> Switch5/1, Switch5/2, Data Type Conversion Inherited/1, Divide1/2, Filtered Derivative (Discrete or Continuous)1/1
  Switch5/1 -> Subtract5/2, Add/1, Data Type Conversion Inherited1/1
  Ipv/1 -> Divide1/1, Filtered Derivative (Discrete or Continuous)/1

== system MicrogridControl/Solar/Solar Plant Integrated1/Detailed/PV Plant & Controller/Controller/MPPT/Solar PV Controller/Variant Subsystem/P&O MPP ==
  Ipv : Inport
  Vpv : Inport  Port=2
  AND1 : Logic  IconShape=distinctive  AllPortsSameDT=off  OutDataTypeStr=boolean
  Add : Sum
  Compare To Zero1 : simulink/Logic and Bit Operations/Compare To Zero  relop=>=  OutDataTypeStr=boolean
  Compare To Zero2 : simulink/Logic and Bit Operations/Compare To Zero  relop=>=  OutDataTypeStr=boolean
  Constant1 : Constant  Value=delV  SampleTime=sampleTime
  Data Type Conversion Inherited : simulink/Signal Attributes/Data Type Conversion Inherited  ConvertRealWorld=Real World Value  DoSatur=off
  Data Type Conversion Inherited1 : simulink/Signal Attributes/Data Type Conversion Inherited  ConvertRealWorld=Real World Value  DoSatur=off
  Filtered Derivative (Discrete or Continuous) : eeGeneralControl/Filtered Derivative (Discrete or Continuous)  K=1  T=tSettling*2  B=inf  A=-inf  minRatio=1  init_option=Inherited from block input  x0=0  Ts=sampleTime
  Filtered Derivative (Discrete or Continuous)1 : eeGeneralControl/Filtered Derivative (Discrete or Continuous)  K=1  T=tSettling*2  B=inf  A=-inf  minRatio=1  init_option=Inherited from block input  x0=0  Ts=sampleTime
  NOR : Logic  Operator=NOR  IconShape=distinctive  AllPortsSameDT=off  OutDataTypeStr=boolean
  OR : Logic  Operator=OR  IconShape=distinctive  AllPortsSameDT=off  OutDataTypeStr=boolean
  Product : Product
  Subtract5 : Sum  Inputs=-+
  Switch4 : Switch  Criteria=u2 ~= 0  SaturateOnIntegerOverflow=off  InputSameDT=off
  Switch5 : Switch  Criteria=u2 > Threshold  SaturateOnIntegerOverflow=off  InputSameDT=off
  start MPPT Voltage : Constant  Value=Vdc  SampleTime=sampleTime
  Vmpp : Outport  VectorParamsAs1DForOutWhenUnconnected=off
  wires:
  Data Type Conversion Inherited1/1 -> Subtract5/1, Add/2
  start MPPT Voltage/1 -> Data Type Conversion Inherited/2
  Data Type Conversion Inherited/1 -> Switch5/3
  Switch4/1 -> Vmpp/1
  Product/1 -> Filtered Derivative (Discrete or Continuous)/1
  Ipv/1 -> Product/1
  [Vinc] -> Switch4/1
  AND1/1 -> OR/1
  Filtered Derivative (Discrete or Continuous)/1 -> Compare To Zero2/1
  Filtered Derivative (Discrete or Continuous)1/1 -> Compare To Zero1/1
  [Vdec] -> Switch4/3
  Subtract5/1 -> [Vdec]  "DEC"
  NOR/1 -> OR/2
  Add/1 -> [Vinc]  "INC"
  Vpv/1 -> Switch5/1, Switch5/2, Data Type Conversion Inherited/1, Filtered Derivative (Discrete or Continuous)1/1, Product/2
  Constant1/1 -> Data Type Conversion Inherited1/2
  Switch5/1 -> Subtract5/2, Add/1, Data Type Conversion Inherited1/1
  Compare To Zero2/1 -> AND1/1, NOR/2
  Compare To Zero1/1 -> AND1/2, NOR/1
  OR/1 -> Switch4/2

== system MicrogridControl/Solar/Solar Plant Integrated1/Detailed/PV Plant & Controller/Controller/Power Reference/Power Reference Controller/PLL & Measurements/Measurement1 ==
  u : Inport
  Lead-Lag (Discrete or Continuous) : eeGeneralControl/Lead-Lag (Discrete or Continuous)  T1=0  T2=1e-3  B=inf  A=-inf  init_option=Inherited from block input  x0=0  Ts=Ts
  Vg : Outport
  wires:
  u/1 -> Lead-Lag (Discrete or Continuous)/1
  Lead-Lag (Discrete or Continuous)/1 -> Vg/1

== system MicrogridControl/Solar/Solar Plant Integrated1/Detailed/PV Plant & Controller/Controller/Power Reference/Power Reference Controller/PLL & Measurements/Measurement2 ==
  u : Inport
  Lead-Lag (Discrete or Continuous) : eeGeneralControl/Lead-Lag (Discrete or Continuous)  T1=0  T2=1e-3  B=inf  A=-inf  init_option=Inherited from block input  x0=0  Ts=Ts
  Vg : Outport
  wires:
  u/1 -> Lead-Lag (Discrete or Continuous)/1
  Lead-Lag (Discrete or Continuous)/1 -> Vg/1

== system MicrogridControl/Solar/Solar Plant Integrated1/Detailed/PV Plant & Controller/Controller/Power Reference/Power Reference Controller/PLL & Measurements/Subsystem ==
  Vabc : Inport
  Iabc : Inport  Port=2
  Demux : Demux  Outputs=3
  Demux1 : Demux  Outputs=3
  Park Transform : eeTransforms/Park Transform  AxisAlignment=Q-axis  PowerInvariant=off
  Park Transform1 : eeTransforms/Park Transform  AxisAlignment=Q-axis  PowerInvariant=off
  Scope : Scope  NumInputPorts=2
      settings: ActiveDisplayYMinimum=0.97158  ActiveDisplayYMaximum=1.00612  DataLoggingVariableName=ScopeData5
  "Sinusoidal Measurement (PLL, Three-Phase)" : eeSinusoidalMeasurementV2/Sinusoidal Measurement (PLL, Three-Phase)  InputFilter=on  InputNormalization=off  Kp_LF=kpPLL  Ki_LF=kiPLL  F0=frequency  Theta0=0  Ts=-1
  Terminator : Terminator
  Terminator1 : Terminator
  mag : Outport
  freq : Outport  Port=2
  angle : Outport  Port=3
  Vd : Outport  Port=4
  Vq : Outport  Port=5
  Id1 : Outport  Port=6
  Iq1 : Outport  Port=7
  wires:
  Iabc/1 -> Park Transform1/1
  Demux1/3 -> Terminator1/1
  Demux1/2 -> Iq1/1
  Demux1/1 -> Id1/1
  Park Transform1/1 -> Demux1/1
  "Sinusoidal Measurement (PLL, Three-Phase)"/3 -> mag/1
  "Sinusoidal Measurement (PLL, Three-Phase)"/1 -> freq/1
  "Sinusoidal Measurement (PLL, Three-Phase)"/2 -> Park Transform/2, Park Transform1/2, angle/1
  Demux/2 -> Vq/1, Scope/2
  Demux/1 -> Vd/1, Scope/1
  Park Transform/1 -> Demux/1
  Vabc/1 -> "Sinusoidal Measurement (PLL, Three-Phase)"/1, Park Transform/1
  Demux/3 -> Terminator/1
